simulink model "mech_spherical_jstick"  (Simulink 7.1)
settings: Solver=ode45  StartTime=0.0  StopTime=10  RelTol=1e-3
undefined symbols (not defined in the file or in its folder): sigbuilder_block
libraries: mblibv1 x16
Description:
  | Spherical Mechanism - Joystick
  | 
  | A spherical mechanism used as a Joystick. The end effector moves on the surface
  | of a sphere. All four revolute axes of the mechanism have to intersect at a single point
  | for the mechanism to have 2 degrees of freedom.
settings Model: Creator=ksanthan  LastModifiedBy=batserve
settings DataIOCC: SaveState=on  SignalLogging=off  StateSaveName=xout_test  OutputTimes=1
settings DebuggingCC: AlgebraicLoopMsg=none  SaveWithParameterizedLinksMsg=none  SignalResolutionControl=TryResolveAllWithWarning  SolverPrmCheckMsg=none
settings GRTTargetCC: TargetFcnLib=ansi_tfl_tmw.mat
settings SimMechanicsCC: WarnOnRedundantConstraints=off  VisOnUpdateDiagram=on  VisDuringSimulation=on

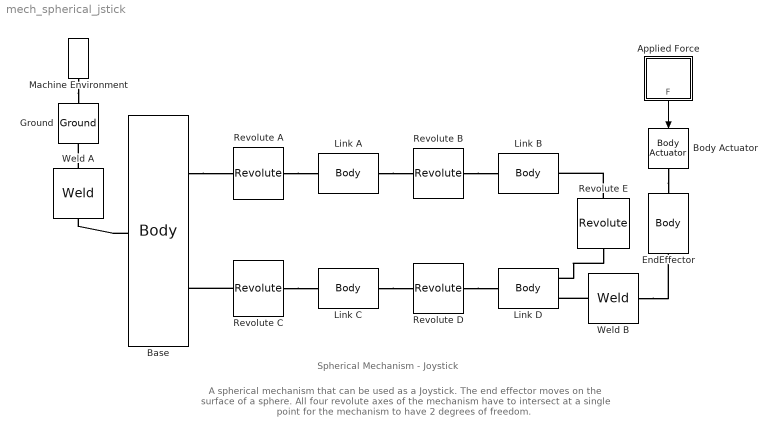
== system mech_spherical_jstick ==
  note: Spherical Mechanism - Joystick
  note: A spherical mechanism that can be used as a Joystick. The end effector moves on the surface
      | of a sphere. All four revolute axes of the mechanism have to intersect at a single point
      | for the mechanism to have 2 degrees of freedom.
  Applied Force : Subsystem  Orientation=down
  Base : mblibv1/Bodies/Body  DialogController=MECH.DynMechDlgSource  PhysicalDomain=mechanical  SubClassName=Unknown  LeftPortType=workingframe  RightPortType=workingframe  LConnTagsString=CS1  RConnTagsString=CS3|CS2  DialogClass=MechanicalBodyBlock  Mass=0.04352  MassUnits=kg  InertiaUnits=kg*m^2  Inertia=[1.5218e-005 -1.1294e-022 0;-1.1294e-022 3.1625e-005 2.8234e-022;0 2.8234e-022 1.7132e-005]  Shape=Joystick10102006_1 - Base-1  ShapeDims=[1 1]  ShapeUnits=m  ShapeUse=false  Density=1  DensityUnits=kg/m^3  DensityUse=false  GraphicsMode=1  BodyColor=[0.5 0.5 0.5]  GraphicsObj=[]  AttachedToCS=1  CG=Right$CG$[0.038 -0.003 -0.03]$WORLD$WORLD$m$[1 0 0;0 1 0;0 0 1]$3x3 Transform$rad$WORLD$false  WorkingFrames=Right$CS3$[-0.01 -0.003 -0.03]$WORLD$WORLD$m$[1 0 0;0 1 0;0 0 1]$3x3 Transform$rad$WORLD$true#Left$CS1$[0 0 0]$WORLD$WORLD$m$[1 0 0;0 1 0;0 0 1]$3x3 Transform$rad$WORLD$true#Right$CS2$[0.038 -0.003 -0.074]$WORLD$WORLD$m$[1 0 0;0 1 0;0 0 1]$3x3 Transform$rad$WORLD$true  CGPos=[0.038 -0.003 -0.03]  CGRot=[1 0 0;0 1 0;0 0 1]  CS0Pos=[]  CS0Rot=[]  CS1Pos=[0 0 0]  CS1Rot=[1 0 0;0 1 0;0 0 1]  CS2Pos=[0.038 -0.003 -0.074]  CS2Rot=[1 0 0;0 1 0;0 0 1]  CS3Pos=[-0.01 -0.003 -0.03]  CS3Rot=[1 0 0;0 1 0;0 0 1]  CS4Pos=[]  CS4Rot=[]  CS5Pos=[]  CS5Rot=[]  CS6Pos=[]  CS6Rot=[]  CS7Pos=[]  CS7Rot=[]  CS8Pos=[]  CS8Rot=[]  CS9Pos=[]  CS9Rot=[]  CS10Pos=[]  CS10Rot=[]  CS11Pos=[]  CS11Rot=[]  CS12Pos=[]  CS12Rot=[]  CS13Pos=[]  CS13Rot=[]  CS14Pos=[]  CS14Rot=[]  CS15Pos=[]  CS15Rot=[]  CS16Pos=[]  CS16Rot=[]  CS17Pos=[]  CS17Rot=[]  CS18Pos=[]  CS18Rot=[]  CS19Pos=[]  CS19Rot=[]  CS20Pos=[]  CS20Rot=[]
  Body Actuator : mblibv1/Sensors &  Actuators/Body Actuator  Orientation=down  DialogController=MECH.DynMechDlgSource  SystemSampleTime=-1  PhysicalDomain=Mechanical  PortType=blob  ActuationStyle=Force  AngleUnits=deg  ArcVelocityUnits=deg/s  ArcAccelerationUnits=deg/s^2  CoordPositionUnits=m  VelocityUnits=m/s  AccelerationUnits=m/s^2  ForceUnits=N  TorqueUnits=N*m  ActiveIO=on  Width=3  DialogClass=MechanicalActuatorBlock  ReferenceFrame=Absolute (World)  Angle=off  CoordPosition=on  Force=on  Torque=off
  EndEffector : mblibv1/Bodies/Body  Orientation=up  DialogController=MECH.DynMechDlgSource  PhysicalDomain=mechanical  SubClassName=Unknown  LeftPortType=workingframe  RightPortType=workingframe  LConnTagsString=CS2  RConnTagsString=CS1  DialogClass=MechanicalBodyBlock  Mass=0.00032  MassUnits=kg  InertiaUnits=kg*m^2  Inertia=[1.1093e-008 -3.0831e-026 -1.3169e-025;-3.0831e-026 1.1093e-008 0;-1.3169e-025 0 8.5333e-010]  Shape=Joystick10102006_1 - EndEffector-1  ShapeDims=[1 1]  ShapeUnits=m  ShapeUse=false  Density=1  DensityUnits=kg/m^3  DensityUse=false  GraphicsMode=1  BodyColor=[0.5 0.5 0.5]  GraphicsObj=[]  AttachedToCS=1  CG=Left$CG$[0.017434 -0.028643 -0.064978]$WORLD$WORLD$m$[0.7801 -0.45592 -0.42845;-0.62565 -0.56848 -0.53423;0 0.68481 -0.72872]$3x3 Transform$rad$WORLD$false  WorkingFrames=Left$CS2$[0.024191 -0.023415 -0.059061]$WORLD$WORLD$m$[1 0 0;0 1 0;0 0 1]$3x3 Transform$rad$WORLD$true#Right$CS1$[0.012501 -0.031597 -0.073635]$WORLD$WORLD$m$[1 0 0;0 1 0;0 0 1]$3x3 Transform$rad$WORLD$true  CGPos=[0.017434 -0.028643 -0.064978]  CGRot=[0.7801 -0.45592 -0.42845;-0.62565 -0.56848 -0.53423;0 0.68481 -0.72872]  CS0Pos=[]  CS0Rot=[]  CS1Pos=[0.012501 -0.031597 -0.073635]  CS1Rot=[1 0 0;0 1 0;0 0 1]  CS2Pos=[0.024191 -0.023415 -0.059061]  CS2Rot=[1 0 0;0 1 0;0 0 1]  CS3Pos=[]  CS3Rot=[]  CS4Pos=[]  CS4Rot=[]  CS5Pos=[]  CS5Rot=[]  CS6Pos=[]  CS6Rot=[]  CS7Pos=[]  CS7Rot=[]  CS8Pos=[]  CS8Rot=[]  CS9Pos=[]  CS9Rot=[]  CS10Pos=[]  CS10Rot=[]  CS11Pos=[]  CS11Rot=[]  CS12Pos=[]  CS12Rot=[]  CS13Pos=[]  CS13Rot=[]  CS14Pos=[]  CS14Rot=[]  CS15Pos=[]  CS15Rot=[]  CS16Pos=[]  CS16Rot=[]  CS17Pos=[]  CS17Rot=[]  CS18Pos=[]  CS18Rot=[]  CS19Pos=[]  CS19Rot=[]  CS20Pos=[]  CS20Rot=[]
  Ground : mblibv1/Bodies/Ground  Orientation=down  DialogController=MECH.DynMechDlgSource  SystemSampleTime=-1  LeftPortType=env  RightPortType=workingframe  PhysicalDomain=Mechanical  DialogClass=GroundBlock  CoordPosition=[0 0 0]  CoordPositionUnits=m  StateVectorMgrId=-1  MachineId=[0 0]  ShowEnvPort=on
  Link A : mblibv1/Bodies/Body  DialogController=MECH.DynMechDlgSource  PhysicalDomain=mechanical  SubClassName=Unknown  LeftPortType=workingframe  RightPortType=workingframe  LConnTagsString=CS2  RConnTagsString=CS3  DialogClass=MechanicalBodyBlock  Mass=0.00095738  MassUnits=kg  InertiaUnits=kg*m^2  Inertia=[1.3208e-007 -1.1613e-007 -1.3908e-024;-1.1613e-007 1.3208e-007 6.2375e-024;-1.3908e-024 6.2375e-024 2.6156e-007]  Shape=Joystick10102006_1 - Part A-1  ShapeDims=[1 1]  ShapeUnits=m  ShapeUse=false  Density=1  DensityUnits=kg/m^3  DensityUse=false  GraphicsMode=1  BodyColor=[0.5 0.5 0.5]  GraphicsObj=[]  AttachedToCS=1  CG=Right$CG$[0.014939 -0.021598 -0.016366]$WORLD$WORLD$m$[1 0 0;0 -0.80649 -0.59124;0 0.59124 -0.80649]$3x3 Transform$rad$WORLD$false  WorkingFrames=Left$CS2$[-0.01 -0.003 -0.03]$WORLD$WORLD$m$[1 0 0;0 1 0;0 0 1]$3x3 Transform$rad$WORLD$true#Right$CS3$[0.038 -0.001387 -0.031182]$WORLD$WORLD$m$[1 0 0;0 1 0;0 0 1]$3x3 Transform$rad$WORLD$true#Right$CS1$[0.002 -0.001387 -0.031182]$WORLD$WORLD$m$[1 0 0;0 1 0;0 0 1]$3x3 Transform$rad$WORLD$false  CGPos=[0.014939 -0.021598 -0.016366]  CGRot=[1 0 0;0 -0.80649 -0.59124;0 0.59124 -0.80649]  CS0Pos=[]  CS0Rot=[]  CS1Pos=[0.002 -0.001387 -0.031182]  CS1Rot=[1 0 0;0 1 0;0 0 1]  CS2Pos=[-0.01 -0.003 -0.03]  CS2Rot=[1 0 0;0 1 0;0 0 1]  CS3Pos=[0.038 -0.001387 -0.031182]  CS3Rot=[1 0 0;0 1 0;0 0 1]  CS4Pos=[]  CS4Rot=[]  CS5Pos=[]  CS5Rot=[]  CS6Pos=[]  CS6Rot=[]  CS7Pos=[]  CS7Rot=[]  CS8Pos=[]  CS8Rot=[]  CS9Pos=[]  CS9Rot=[]  CS10Pos=[]  CS10Rot=[]  CS11Pos=[]  CS11Rot=[]  CS12Pos=[]  CS12Rot=[]  CS13Pos=[]  CS13Rot=[]  CS14Pos=[]  CS14Rot=[]  CS15Pos=[]  CS15Rot=[]  CS16Pos=[]  CS16Rot=[]  CS17Pos=[]  CS17Rot=[]  CS18Pos=[]  CS18Rot=[]  CS19Pos=[]  CS19Rot=[]  CS20Pos=[]  CS20Rot=[]
  Link B : mblibv1/Bodies/Body  DialogController=MECH.DynMechDlgSource  PhysicalDomain=mechanical  SubClassName=Unknown  LeftPortType=workingframe  RightPortType=workingframe  LConnTagsString=CS2  RConnTagsString=CS3  DialogClass=MechanicalBodyBlock  Mass=0.00085171  MassUnits=kg  InertiaUnits=kg*m^2  Inertia=[9.2815e-008 -8.161e-008 2.0937e-024;-8.161e-008 9.4305e-008 -2.2187e-024;2.0937e-024 -2.2187e-024 1.8479e-007]  Shape=Joystick10102006_1 - Part B-1  ShapeDims=[1 1]  ShapeUnits=m  ShapeUse=false  Density=1  DensityUnits=kg/m^3  DensityUse=false  GraphicsMode=1  BodyColor=[0.5 0.5 0.5]  GraphicsObj=[]  AttachedToCS=1  CG=Right$CG$[0.029159 -0.03051 -0.032951]$WORLD$WORLD$m$[0 -0.42845 -0.90356;0.80649 -0.53423 0.25332;-0.59124 -0.72872 0.34554]$3x3 Transform$rad$WORLD$false  WorkingFrames=Left$CS2$[0.038 -0.001387 -0.031182]$WORLD$WORLD$m$[1 0 0;0 1 0;0 0 1]$3x3 Transform$rad$WORLD$true#Right$CS3$[0.038857 -0.0019316 -0.028543]$WORLD$WORLD$m$[1 0 0;0 1 0;0 0 1]$3x3 Transform$rad$WORLD$true#Right$CS1$[0.038857 -0.027739 -0.0096228]$WORLD$WORLD$m$[1 0 0;0 1 0;0 0 1]$3x3 Transform$rad$WORLD$false  CGPos=[0.029159 -0.03051 -0.032951]  CGRot=[0 -0.42845 -0.90356;0.80649 -0.53423 0.25332;-0.59124 -0.72872 0.34554]  CS0Pos=[]  CS0Rot=[]  CS1Pos=[0.038857 -0.027739 -0.0096228]  CS1Rot=[1 0 0;0 1 0;0 0 1]  CS2Pos=[0.038 -0.001387 -0.031182]  CS2Rot=[1 0 0;0 1 0;0 0 1]  CS3Pos=[0.038857 -0.0019316 -0.028543]  CS3Rot=[1 0 0;0 1 0;0 0 1]  CS4Pos=[]  CS4Rot=[]  CS5Pos=[]  CS5Rot=[]  CS6Pos=[]  CS6Rot=[]  CS7Pos=[]  CS7Rot=[]  CS8Pos=[]  CS8Rot=[]  CS9Pos=[]  CS9Rot=[]  CS10Pos=[]  CS10Rot=[]  CS11Pos=[]  CS11Rot=[]  CS12Pos=[]  CS12Rot=[]  CS13Pos=[]  CS13Rot=[]  CS14Pos=[]  CS14Rot=[]  CS15Pos=[]  CS15Rot=[]  CS16Pos=[]  CS16Rot=[]  CS17Pos=[]  CS17Rot=[]  CS18Pos=[]  CS18Rot=[]  CS19Pos=[]  CS19Rot=[]  CS20Pos=[]  CS20Rot=[]
  Link C : mblibv1/Bodies/Body  Orientation=left  DialogController=MECH.DynMechDlgSource  PhysicalDomain=mechanical  SubClassName=Unknown  LeftPortType=workingframe  RightPortType=workingframe  LConnTagsString=CS2  RConnTagsString=CS3  DialogClass=MechanicalBodyBlock  Mass=0.00085171  MassUnits=kg  InertiaUnits=kg*m^2  Inertia=[9.2815e-008 -8.161e-008 2.0937e-024;-8.161e-008 9.4305e-008 -2.2187e-024;2.0937e-024 -2.2187e-024 1.8479e-007]  Shape=Joystick10102006_1 - Part B-2  ShapeDims=[1 1]  ShapeUnits=m  ShapeUse=false  Density=1  DensityUnits=kg/m^3  DensityUse=false  GraphicsMode=1  BodyColor=[0.5 0.5 0.5]  GraphicsObj=[]  AttachedToCS=1  CG=Right$CG$[0.054098 -0.015911 -0.050442]$WORLD$WORLD$m$[0 0.7801 0.62565;0 -0.62565 0.7801;1 0 0]$3x3 Transform$rad$WORLD$false  WorkingFrames=Left$CS2$[0.03644 -0.0017487 -0.03]$WORLD$WORLD$m$[1 0 0;0 1 0;0 0 1]$3x3 Transform$rad$WORLD$true#Right$CS3$[0.038 -0.003 -0.074]$WORLD$WORLD$m$[1 0 0;0 1 0;0 0 1]$3x3 Transform$rad$WORLD$true  CGPos=[0.054098 -0.015911 -0.050442]  CGRot=[0 0.7801 0.62565;0 -0.62565 0.7801;1 0 0]  CS0Pos=[]  CS0Rot=[]  CS1Pos=[]  CS1Rot=[]  CS2Pos=[0.03644 -0.0017487 -0.03]  CS2Rot=[1 0 0;0 1 0;0 0 1]  CS3Pos=[0.038 -0.003 -0.074]  CS3Rot=[1 0 0;0 1 0;0 0 1]  CS4Pos=[]  CS4Rot=[]  CS5Pos=[]  CS5Rot=[]  CS6Pos=[]  CS6Rot=[]  CS7Pos=[]  CS7Rot=[]  CS8Pos=[]  CS8Rot=[]  CS9Pos=[]  CS9Rot=[]  CS10Pos=[]  CS10Rot=[]  CS11Pos=[]  CS11Rot=[]  CS12Pos=[]  CS12Rot=[]  CS13Pos=[]  CS13Rot=[]  CS14Pos=[]  CS14Rot=[]  CS15Pos=[]  CS15Rot=[]  CS16Pos=[]  CS16Rot=[]  CS17Pos=[]  CS17Rot=[]  CS18Pos=[]  CS18Rot=[]  CS19Pos=[]  CS19Rot=[]  CS20Pos=[]  CS20Rot=[]
  Link D : mblibv1/Bodies/Body  Orientation=left  DialogController=MECH.DynMechDlgSource  PhysicalDomain=mechanical  SubClassName=Unknown  LeftPortType=workingframe  RightPortType=workingframe  LConnTagsString=CS2|CS4  RConnTagsString=CS3  DialogClass=MechanicalBodyBlock  Mass=0.00095738  MassUnits=kg  InertiaUnits=kg*m^2  Inertia=[1.3208e-007 -1.1613e-007 -9.1538e-025;-1.1613e-007 1.3208e-007 6.1622e-024;-9.1538e-025 6.1622e-024 2.6156e-007]  Shape=Joystick10102006_1 - Part A-2  ShapeDims=[1 1]  ShapeUnits=m  ShapeUse=false  Density=1  DensityUnits=kg/m^3  DensityUse=false  GraphicsMode=1  BodyColor=[0.5 0.5 0.5]  GraphicsObj=[]  AttachedToCS=1  CG=Right$CG$[0.046109 -0.029748 -0.046805]$WORLD$WORLD$m$[-0.7801 -0.42845 -0.45592;0.62565 -0.53423 -0.56848;0 -0.72872 0.68481]$3x3 Transform$rad$WORLD$false  WorkingFrames=Left$CS2$[0.038857 -0.0019316 -0.028543]$WORLD$WORLD$m$[1 0 0;0 1 0;0 0 1]$3x3 Transform$rad$WORLD$true#Right$CS3$[0.03644 -0.0017487 -0.03]$WORLD$WORLD$m$[1 0 0;0 1 0;0 0 1]$3x3 Transform$rad$WORLD$true#Left$CS4$[0.024191 -0.023415 -0.059061]$WORLD$WORLD$m$[1 0 0;0 1 0;0 0 1]$3x3 Transform$rad$WORLD$true  CGPos=[0.046109 -0.029748 -0.046805]  CGRot=[-0.7801 -0.42845 -0.45592;0.62565 -0.53423 -0.56848;0 -0.72872 0.68481]  CS0Pos=[]  CS0Rot=[]  CS1Pos=[]  CS1Rot=[]  CS2Pos=[0.038857 -0.0019316 -0.028543]  CS2Rot=[1 0 0;0 1 0;0 0 1]  CS3Pos=[0.03644 -0.0017487 -0.03]  CS3Rot=[1 0 0;0 1 0;0 0 1]  CS4Pos=[0.024191 -0.023415 -0.059061]  CS4Rot=[1 0 0;0 1 0;0 0 1]  CS5Pos=[]  CS5Rot=[]  CS6Pos=[]  CS6Rot=[]  CS7Pos=[]  CS7Rot=[]  CS8Pos=[]  CS8Rot=[]  CS9Pos=[]  CS9Rot=[]  CS10Pos=[]  CS10Rot=[]  CS11Pos=[]  CS11Rot=[]  CS12Pos=[]  CS12Rot=[]  CS13Pos=[]  CS13Rot=[]  CS14Pos=[]  CS14Rot=[]  CS15Pos=[]  CS15Rot=[]  CS16Pos=[]  CS16Rot=[]  CS17Pos=[]  CS17Rot=[]  CS18Pos=[]  CS18Rot=[]  CS19Pos=[]  CS19Rot=[]  CS20Pos=[]  CS20Rot=[]
  Machine Environment : mblibv1/Bodies/Machine Environment  Tag=Factory ground  Orientation=down  DialogController=MECH.DialogSource  SystemSampleTime=-1  PortType=env  PhysicalDomain=Mechanical  DialogTemplateClass=MECH.MachineEnvironment  SyncWhenCopied=off  Gravity=[0 0 0]  GravityUnits=m/s^2  GravityAsSignal=off  Dimensionality=Auto-detect  AnalysisType=Forward dynamics  LinearAssemblyTolerance=1e-3  LinearAssemblyToleranceUnits=m  AngularAssemblyTolerance=1e-3  AngularAssemblyToleranceUnits=rad  ConstraintSolverType=Stabilizing  ConstraintRelTolerance=1e-4  ConstraintAbsTolerance=1e-4  UseRobustSingularityHandling=off  RedundancyAnalysisToleranceType=Specify tolerance  RedundancyAnalysisTolerance=1e-6  StatePerturbationType=Fixed  PerturbationSize=1e-5  VisualizeMachine=on
  Revolute A : mblibv1/Joints/Revolute  DialogController=MECH.DynMechDlgSource  PhysicalDomain=mechanical  SubClassName=Unknown  LeftPortType=blob  RightPortType=blob  LConnTagsString=__newl0  RConnTagsString=__newr0  NumSAPorts=0  CutJoint=off  MarkAsCut=off  Primitives=prismatic  PrimitiveProps=R1$World$[1 0 0]$revolute  DialogClass=JointBlock  R1Axis=[1 0 0]
  Revolute B : mblibv1/Joints/Revolute  DialogController=MECH.DynMechDlgSource  PhysicalDomain=mechanical  SubClassName=Unknown  LeftPortType=blob  RightPortType=blob  LConnTagsString=__newl0  RConnTagsString=__newr0  NumSAPorts=0  CutJoint=on  MarkAsCut=off  Primitives=prismatic  PrimitiveProps=R1$World$[0 -0.80649 0.59124]$revolute  DialogClass=JointBlock  R1Axis=[0 -0.80649 0.59124]
  Revolute C : mblibv1/Joints/Revolute  DialogController=MECH.DynMechDlgSource  PhysicalDomain=mechanical  SubClassName=Unknown  LeftPortType=blob  RightPortType=blob  LConnTagsString=__newl0  RConnTagsString=__newr0  NumSAPorts=0  CutJoint=off  MarkAsCut=off  Primitives=prismatic  PrimitiveProps=R1$World$[0 0 1]$revolute  DialogClass=JointBlock  R1Axis=[0 0 1]
  Revolute D : mblibv1/Joints/Revolute  Orientation=left  DialogController=MECH.DynMechDlgSource  PhysicalDomain=mechanical  SubClassName=Unknown  LeftPortType=blob  RightPortType=blob  LConnTagsString=__newl0  RConnTagsString=__newr0  NumSAPorts=0  CutJoint=off  MarkAsCut=off  Primitives=prismatic  PrimitiveProps=R1$World$[0.7801 -0.62565 0]$revolute  DialogClass=JointBlock  R1Axis=[0.7801 -0.62565 0]
  Revolute E : mblibv1/Joints/Revolute  Orientation=down  DialogController=MECH.DynMechDlgSource  PhysicalDomain=mechanical  SubClassName=Unknown  LeftPortType=blob  RightPortType=blob  LConnTagsString=__newl0  RConnTagsString=__newr0  NumSAPorts=0  CutJoint=off  MarkAsCut=off  Primitives=prismatic  PrimitiveProps=R1$World$[-0.42845 -0.53423 -0.72872]$revolute  DialogClass=JointBlock  R1Axis=[-0.42845 -0.53423 -0.72872]
  Weld A : mblibv1/Joints/Weld  Orientation=down  DialogController=MECH.DynMechDlgSource  PhysicalDomain=mechanical  SubClassName=Unknown  LeftPortType=blob  RightPortType=blob  LConnTagsString=__newl0  RConnTagsString=__newr0  NumSAPorts=0  CutJoint=off  MarkAsCut=off  Primitives=weld  PrimitiveProps=W$WORLD$[0 0 0]$weld  DialogClass=JointBlock  WAxis=[0 0 0]
  Weld B : mblibv1/Joints/Weld  DialogController=MECH.DynMechDlgSource  PhysicalDomain=mechanical  SubClassName=Unknown  LeftPortType=blob  RightPortType=blob  LConnTagsString=__newl0  RConnTagsString=__newr0  NumSAPorts=0  CutJoint=off  MarkAsCut=off  Primitives=weld  PrimitiveProps=W$WORLD$[1 1 1]$weld  DialogClass=JointBlock  WAxis=[1 1 1]
  wires:
  Applied Force/1(F) -> Body Actuator/1
  connections:
  Revolute C/LConn1 -- Base/RConn2
  Revolute A/RConn1 -- Link A/LConn1
  Revolute E/RConn1 -- Link D/LConn1
  Weld B/RConn1 -- EndEffector/LConn1
  Weld A/LConn1 -- Ground/RConn1
  Revolute D/LConn1 -- Link D/RConn1
  Revolute E/LConn1 -- Link B/RConn1
  Revolute B/RConn1 -- Link B/LConn1
  Base/LConn1 -- Weld A/RConn1
  Base/RConn1 -- Revolute A/LConn1
  Link A/RConn1 -- Revolute B/LConn1
  Revolute C/RConn1 -- Link C/RConn1
  Link C/LConn1 -- Revolute D/RConn1
  Weld B/LConn1 -- Link D/LConn2
  Body Actuator/RConn1 -- EndEffector/RConn1
  Machine Environment/RConn1 -- Ground/LConn1

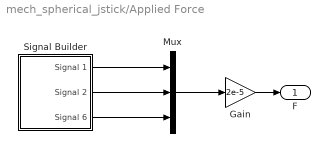
== system mech_spherical_jstick/Applied Force ==
  Gain : Gain  Gain=2e-5  ParameterDataType=sfix(16)  ParameterScaling=2^0  OutDataType=sfix(16)  OutScaling=2^0
  Mux : Mux  Inputs=3
  Signal Builder : Subsystem  Tag=STV Subsys  LoadFcn=sigbuilder_block('load');  StartFcn=sigbuilder_block('start');  StopFcn=sigbuilder_block('stop');  ClipboardFcn=sigbuilder_block('clipboard');  mask(Sigbuilder block){}
      mask help: Sigbuilder GUI
      mask init:
      | if ~strcmp(get_param(bdroot(gcbh),'SimulationStatus'),'stopped') tuvar = sigbuilder_block('maskInit'); end
      settings: CopyFcn=sigbuilder_block('copy');  DeleteFcn=sigbuilder_block('delete');  ModelCloseFcn=sigbuilder_block('modelClose');  PreSaveFcn=sigbuilder_block('preSave');  NameChangeFcn=sigbuilder_block('namechange');  OpenFcn=sigbuilder_block('open',[3 22.5 1434 791.25 ]);  CloseFcn=sigbuilder_block('close');
      mask Display: plot(0,0,100,100,[10,10,40,40,10],[80,20,20,80,80],[40,10],[50,50], [40,27,10],[65,72,56],[40,25,25,10],[28,28,43,43]);
  F : Outport  OutDataType=sfix(16)  OutScaling=2^0
  wires:
  Signal Builder/1(Signal 1) -> Mux/1
  Signal Builder/2(Signal 2) -> Mux/2
  Signal Builder/3(Signal 6) -> Mux/3
  Mux/1 -> Gain/1
  Gain/1 -> F/1

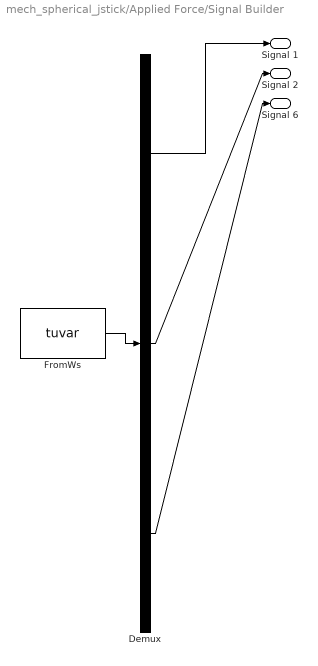
== system mech_spherical_jstick/Applied Force/Signal Builder ==
  Demux : Demux  Tag=STV Demux  Outputs=3
  FromWs : FromWorkspace  Tag=STV FromWs  VariableName=tuvar  SampleTime=0  SigBuilderData=DataTag0  VnvData=DataTag1
      SigBuilderData=|
      | channels(1).label = 'Signal 1'
      | channels(1).allXData = {[0 1.49 3.47 3.47 4.01 6 6 7.5 7.5 10]}
      | channels(1).allYData = {[0 0 0 1 1 1 -1 -1 0 0]}
      | channels(2).label = 'Signal 2'
      | channels(2).allXData = {[0 1.48 4.01 5.01 10]}
      | channels(2).allYData = {[0 0 0 0 0]}
      | channels(3).label = 'Signal 6'
      | channels(3).allXData = {[0 2 2 4 4 6.99 6.99 10]}
      | channels(3).allYData = {[1 1 -1 -1 0 0 0.98 0.98]}
      | common.afterFinalStr = 'Extrapolate'
      | common.sampleTime = 0
      | dataSet.timeRange = [0 10]
      | dataSet.name = 'Group 1'
  Signal 1 : Outport  Tag=STV Outport  OutDataType=sfix(16)  OutScaling=2^0
  Signal 2 : Outport  Tag=STV Outport  Port=2  OutDataType=sfix(16)  OutScaling=2^0
  Signal 6 : Outport  Tag=STV Outport  Port=3  OutDataType=sfix(16)  OutScaling=2^0
  wires:
  Demux/1 -> Signal 1/1
  FromWs/1 -> Demux/1
  Demux/2 -> Signal 2/1
  Demux/3 -> Signal 6/1
